simulink model "comp_hyb1206"  (R2018a)
settings: Solver=ode45  StartTime=0.0  StopTime=10  RelTol=1e-3  EnableMultiTasking=on
undefined symbols (not defined in the file or in its folder): Ion, Lithium, sigbuilder_block
libraries: powerlib x26, powerlib_meascontrol x7, powerlib_extras x2, electricdrivelib x1, re_lib x1
settings Model: Creator=Amr Saleh  LastModifiedBy=CC
settings DataIOCC: LimitDataPoints=on  SaveFormat=Array
settings OptimizationCC: LifeSpan=inf
settings DebuggingCC: SolverPrmCheckMsg=warning  SFUnexpectedBacktrackingDiag=warning  SFNoUnconditionalDefaultTransitionDiag=warning  SFExecutionAtInitializationDiag=none
settings HardwareCC: ProdBitPerPointer=32  ProdBitPerSizeT=32  ProdBitPerPtrDiffT=32  ProdLargestAtomicFloat=None  ProdIntDivRoundTo=Undefined  ProdEndianess=Unspecified  ProdWordSize=32  ProdHWDeviceType=32-bit Generic
settings ModelReferenceCC: PropagateSignalLabelsOutOfModel=off
settings CodeAppCC: StateflowObjectComments=on
settings GRTTargetCC: TargetLangStandard=C89/C90 (ANSI)  GeneratePreprocessorConditionals=Disable all
settings ConfigComp: CovMetricSettings=dw  CovHtmlReporting=on  CovSaveCumulativeToWorkspaceVar=on  CovSaveSingleToWorkspaceVar=on  CovExternalEMLEnable=off  CovSFcnEnable=off

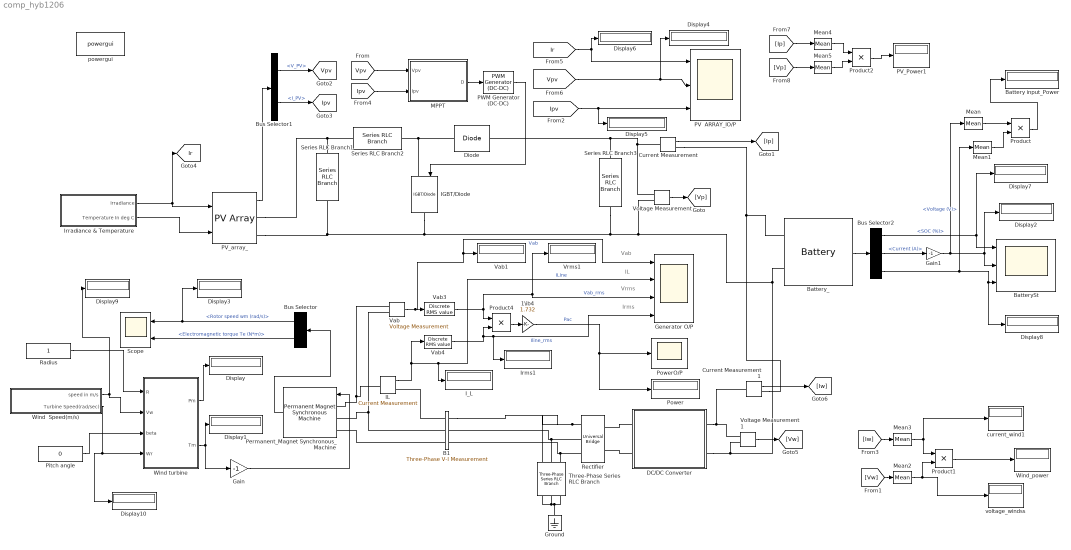
== system comp_hyb1206 ==
  note: Vrms
  note: Vab
  note: IL
  note: Irms
  1\ib4 : Gain  Gain=1.732  SaturateOnIntegerOverflow=on  OutDataTypeStr=Inherit: Same as input  ParamDataTypeStr=Inherit: Same as input
  B1 : powerlib/Measurements/Three-Phase V-I Measurement  VoltageMeasurement=phase-to-ground  SetLabelV=on  LabelV=Vabc_B1  Vpu=off  VpuLL=off  CurrentMeasurement=yes  SetLabelI=on  LabelI=Iabc_B1  Ipu=off  Pbase=100e6  Vbase=500e3  OutputType=Magnitude  PhasorSimulation=off  PSBequivalent=0
  Battery input_Power : Display
  BatterySt : Scope  NumInputPorts=3
  Battery_ : electricdrivelib/Extra Sources/Battery  BatType=Lithium-Ion  ShowTempParam=off  ThermalPreset=no  ShowAgeParam=off  NomV=240  NomQ=100  SOC=49.001  Batt_Tr=30  PresetModel=on  MaxQ=100  MinV=180  FullV=279.3569  Dis_rate=43.4783  R=0.024  Normal_OP=90.4348  expZone="[259.2926      4.913043]"  current=[6.5 13 32.5]  Units=Time  Tci=20  NomT=20  T2=-30  MaxQ2=4.8  FullV2=7.1  Normal_OP2=5.655  expZone2="[6.58           1]"  Rca=0.6  ti=2000  Dp=0  Neq0=0  Tsim=1e6  Ta1=25  Qeol=5.4*0.9  Reol=0.013333*1.2  Char_age=[2.3478, 3]  Dis_age=[2.3478, 10]  N1=1500  N2=10500  N3=1000  N4=1400  Ta2=45  N5=950
  Bus Selector : BusSelector  OutputSignals=Rotor speed wm (rad/s),Electromagnetic torque Te (N*m)
  Bus Selector1 : BusSelector  OutputSignals=V_PV,I_PV
  Bus Selector2 : BusSelector  OutputSignals=SOC (%),Current (A),Voltage (V)
  Current Measurement : powerlib/Measurements/Current Measurement  PhasorSimulation=off  OutputType=Complex  PSBequivalent=0
  Current Measurement1 : powerlib/Measurements/Current Measurement  PhasorSimulation=off  OutputType=Complex  PSBequivalent=0
  DC/DC Converter : Subsystem
  Diode : powerlib/Power Electronics/Diode  Ron=0.001  Lon=0  Vf=0.8  IC=0  UseSnubber=0  Rs=500  Cs=250e-9  Measurements=off
  Display{,1..10} (11 alike) : Display
      Display10 settings: Decimation=2
  Gain : Gain  Gain=-1
  Gain1 : Gain  Gain=-1
  Generator O/P : Scope  NumInputPorts=4
  Ground : powerlib/Elements/Ground  LConnTagsString=a
  IGBT/Diode : powerlib/Power Electronics/IGBT//Diode  Ron=1e-3  Rs=1e5  Cs=inf  Measurements=off
  IL : powerlib/Measurements/Current Measurement  PhasorSimulation=off  OutputType=Complex  PSBequivalent=0
  I_L : Display
      settings: SampleTime=1e-3
  Irms1 : Display
      settings: SampleTime=1e-3
  Irradiance & Temperature : Subsystem  Tag=STV Subsys  LoadFcn=sigbuilder_block('load');  StartFcn=sigbuilder_block('start');  StopFcn=sigbuilder_block('stop');  ClipboardFcn=sigbuilder_block('clipboard');  mask(Sigbuilder block){tuvar=[0:10]}
      mask help: Simulink:masks:SigbuilderBlock_MD
      mask init:
      | if ~strcmp(get_param(bdroot(gcbh),'SimulationStatus'),'stopped') tuvar = sigbuilder_block('maskInit'); end
      settings: CopyFcn=sigbuilder_block('copy');  DeleteFcn=sigbuilder_block('delete');  ModelCloseFcn=sigbuilder_block('modelClose');  PreSaveFcn=sigbuilder_block('preSave');  PauseFcn=sigbuilder_block('pause');  ContinueFcn=sigbuilder_block('continue');  NameChangeFcn=sigbuilder_block('namechange');  OpenFcn=sigbuilder_block('open',[437.4 186 550.8 400.2 ]);  CloseFcn=sigbuilder_block('close');
      mask Display: plot(0, 0, 100, 100,[2, 2, 32, 32, 2], [68, 8, 8, 68, 68],[32, 2], [38, 38], [32, 19, 2],[53, 60, 44], [32, 17, 17, 2],[16, 16, 31, 31]);txt = getActiveGroup(gcbh);text(2, 100, txt,'verticalAlignment', 'top');
  MPPT : MATLAB Function  TreatAsAtomicUnit=on
  Mean{,1..5} (6 alike) : powerlib_meascontrol/Measurements/Mean  Freq=60  Vinit=0  Ts=0
  PV  ARRAY_lO/P : Scope  NumInputPorts=3
  PV_Power1 : Display
  PV_array_ : re_lib/Solar/PV Array  Npar=2  Nser=5  PlotType=array @ 1000 W/m2 & specified temperatures  S_vec="[ 1000  500  100 ]"  Temp_C_vec="[ 45 25  ]"  ModuleName=User-defined  PlotWhenSelected=off  Pm=200.112  Ncell=60  Voc=32.9  Isc=8.21  Vm=26.4  Im=7.58  beta_Voc_pc=-0.35339  alpha_Isc_pc=0.055349  beta_Voc=-0.11627  alpha_Isc=0.0045442  IL=8.232  I0=2.1756e-10  nI=0.87743  Rsh=123.7196  Rs=0.3317  BAL=on  Tc=1e-6  Tfilter=5e-5
  PWM Generator (DC-DC) : powerlib_meascontrol/Pulse & Signal Generators/PWM Generator (DC-DC)  Fsw=5000  Ts=10e-6
  Permanent_Magnet Synchronous_Machine : powerlib/Machines/Permanent Magnet Synchronous Machine  NbPhases=3  FluxDistribution=Sinusoidal  RotorType=Round  MechanicalLoad=Torque Tm  PresetModel=No  ShowDetailedParameters=on  MeasurementBus=off  Resistance=0.0485  Inductance=8.5e-3  dqInductances=[8.5e-3,8.5e-3]  La=0.000395  MachineConstant=Flux linkage established by magnets (V.s)  Flux=0.433  VoltageCst=392.6876  TorqueCst=3.2475  Flat=120  Mechanical=[0.01197 0.001189 5]  PolePairs=4  InitialConditions=[0,0, 0,0]  InitialConditions5ph=[0 0 0 0 0 0]  TsPowergui=0  TsBlock=-1  RefAngle=90 degrees behind phase A axis (modified Park)
      settings: SourceProductName=Simscape Power Systems
  Pitch angle : Constant  Value=0
  Power : Display
      settings: SampleTime=1e-3
  PowerO/P : Scope
  Product : Product
  Product1 : Product
  Product2 : Product
  Product4 : Product  RndMeth=Zero
  Radius : Constant
  Rectifier : powerlib/Power Electronics/Universal Bridge  Arms=3  SnubberResistance=1e5  SnubberCapacitance=inf  Device=Diodes  Ron=1e-3  Lon=0  ForwardVoltages="[  0  0  ]"  ForwardVoltage=0  GTOparameters=[ 10e-6 , 20e-6 ]  IGBTparameters=[ 1e-6 , 2e-6 ]  Measurements=None  Measurements_2=None  converterType=Rectifier
  Scope : Scope  NumInputPorts=2
  Series RLC Branch1 : powerlib/Elements/Series RLC Branch  LConnTagsString=__new0  RConnTagsString=__new0  BranchType=RC  Resistance=1e-4  Inductance=1e-3  SetiL0=off  InitialCurrent=0  Capacitance=100e-6  Setx0=off  InitialVoltage=0  Measurements=None
  Series RLC Branch2 : powerlib/Elements/Series RLC Branch  LConnTagsString=__new0  RConnTagsString=__new0  BranchType=RL  Resistance=0.1  Inductance=5e-3  SetiL0=off  InitialCurrent=0  Capacitance=100e-6  Setx0=off  InitialVoltage=0  Measurements=None
  Series RLC Branch3 : powerlib/Elements/Series RLC Branch  LConnTagsString=__new0  RConnTagsString=__new0  BranchType=RC  Resistance=1e-4  Inductance=1e-3  SetiL0=off  InitialCurrent=0  Capacitance=3300e-6  Setx0=off  InitialVoltage=0  Measurements=None
  Three-Phase Series RLC Branch : powerlib/Elements/Three-Phase Series RLC Branch  LConnTagsString=A|B|C  RConnTagsString=A|B|C  BranchType=C  Resistance=25  Inductance=1e-3  Capacitance=10e-6  Measurements=None
  Vab : powerlib/Measurements/Voltage Measurement  PhasorSimulation=off  OutputType=Complex  PSBequivalent=0
  Vab1 : Display
      settings: SampleTime=1e-3
  Vab3 : powerlib_extras/Discrete Measurements/Discrete  RMS value  Freq=50  Mag_Init=0  Ts=20e-6
  Vab4 : powerlib_extras/Discrete Measurements/Discrete  RMS value  Freq=50  Mag_Init=0  Ts=20e-6
  Voltage Measurement : powerlib/Measurements/Voltage Measurement  PhasorSimulation=off  OutputType=Complex  PSBequivalent=0
  Voltage Measurement1 : powerlib/Measurements/Voltage Measurement  PhasorSimulation=off  OutputType=Complex  PSBequivalent=0
  Vrms1 : Display
      settings: SampleTime=1e-3
  Wind  Speed(m/s) : Subsystem  Tag=STV Subsys  LoadFcn=sigbuilder_block('load');  StartFcn=sigbuilder_block('start');  StopFcn=sigbuilder_block('stop');  ClipboardFcn=sigbuilder_block('clipboard');  mask(Sigbuilder block){tuvar=[0:10]}
      mask help: Simulink:masks:SigbuilderBlock_MD
      mask init:
      | if ~strcmp(get_param(bdroot(gcbh),'SimulationStatus'),'stopped') tuvar = sigbuilder_block('maskInit'); end
      settings: CopyFcn=sigbuilder_block('copy');  DeleteFcn=sigbuilder_block('delete');  ModelCloseFcn=sigbuilder_block('modelClose');  PreSaveFcn=sigbuilder_block('preSave');  PauseFcn=sigbuilder_block('pause');  ContinueFcn=sigbuilder_block('continue');  NameChangeFcn=sigbuilder_block('namechange');  OpenFcn=sigbuilder_block('open',[330.6 139.8 550.8 400.2 ]);  CloseFcn=sigbuilder_block('close');
      mask Display: plot(0, 0, 100, 100,[2, 2, 32, 32, 2], [68, 8, 8, 68, 68],[32, 2], [38, 38], [32, 19, 2],[53, 60, 44], [32, 17, 17, 2],[16, 16, 31, 31]);txt = getActiveGroup(gcbh);text(2, 100, txt,'verticalAlignment', 'top');
  Wind turbine : Subsystem
  Wind_power : Display
  current_wind1 : Display
  powergui : powerlib/powergui  Priority=1  SimulationMode=Discrete  SampleTime=1e-6  frequency=60  Iterations=50  frequencyindice=0  Pbase=100e6  ErrMax=1e-4  UnitsV=kV  UnitsW=MW  buscounter=0  FunctionMessages=off  echomessages=off  EnableUseOfTLC=off  CurrentSourceSwitches=off  DisableSnubberDevices=off  DisableRonSwitches=off  DisableVfSwitches=off  DisplayEquations=off  SolverType=Tustin/Backward Euler (TBE)  Interpol=off  ExternalGateDelay=off  methode=off  Ts=100  x0status=blocks  SPID=on  SwTol=0  HookPort=off  RestoreLinks=warning  ResistiveCurrentMeasurement=off  Frange=[0:2:500]  Ylog=off  Xlog=on  ShowGrid=off  save=off  variable=ZData  structure=0  ZoomFFT=off  StartTime=0.0  cycles=1  DisplayStyle=1  fundamental=60  FreqAxis=off  MaxFrequency=1000  frequencyindicesteady=1  RmsSteady=1  display=off
  voltage_windss : Display
  tag scope: Ipv=global, Ir=global, Vpv=global
  wires:
  Radius/1 -> Wind turbine/1(R)
  Wind  Speed(m/s)/1(speed in m/s) -> Display9/1, Wind turbine/2(Vw)
  Pitch angle/1 -> Wind turbine/3(beta)
  Wind  Speed(m/s)/2(Turbine Speed(rad/sec)) -> Display10/1, Wind turbine/4(Wr)
  Wind turbine/1(Pm) -> Display/1
  Vab4/1 -> Product4/2, Irms1/1, Generator O/P/4  "Iline_rms"
  1\ib4/1 -> Power/1, PowerO/P/1  "Pac"
  Product4/1 -> 1\ib4/1
  IL/1 -> I_L/1, Generator O/P/2, Vab4/1  "ILine"
  Vab/1 -> Vab1/1, Generator O/P/1, Vab3/1  "Vab"
  Vab3/1 -> Vrms1/1, Generator O/P/3, Product4/1  "Vab_rms"
  Wind turbine/2(Tm) -> Gain/1, Display1/1
  Gain/1 -> Permanent_Magnet Synchronous_Machine/1
  Permanent_Magnet Synchronous_Machine/1 -> Bus Selector/1
  Bus Selector/1 -> Display3/1, Scope/1  "<Rotor speed wm (rad/s)>"
  Bus Selector/2 -> Scope/2  "<Electromagnetic torque Te (N*m)>"
  [Vpv] -> MPPT/1(Vpv)
  Bus Selector1/2 -> [Ipv]  "<I_PV>"
  [Vpv] -> Display4/1, PV  ARRAY_lO/P/2
  PV_array_/1 -> Bus Selector1/1
  PWM Generator (DC-DC)/1 -> IGBT/Diode/1
  Bus Selector1/1 -> [Vpv]  "<V_PV>"
  MPPT/1(D) -> PWM Generator (DC-DC)/1
  [Ipv] -> Display5/1, PV  ARRAY_lO/P/3
  [Ipv] -> MPPT/2(Ipv)
  Battery_/1 -> Bus Selector2/1
  Bus Selector2/1 -> BatterySt/1, Display7/1  "<SOC (%)>"
  Bus Selector2/2 -> Gain1/1  "<Current (A)>"
  Bus Selector2/3 -> Mean1/1, Display8/1, BatterySt/3  "<Voltage (V)>"
  [Ir] -> PV  ARRAY_lO/P/1, Display6/1
  Gain1/1 -> Mean/1, Display2/1, BatterySt/2
  Mean/1 -> Product/1
  Mean1/1 -> Product/2
  Product/1 -> Battery input_Power/1
  Voltage Measurement/1 -> [Vp]
  Current Measurement/1 -> [Ip]
  [Ip] -> Mean4/1
  [Vp] -> Mean5/1
  Mean4/1 -> Product2/1
  Mean5/1 -> Product2/2
  Product2/1 -> PV_Power1/1
  Voltage Measurement1/1 -> [Vw]
  Current Measurement1/1 -> [Iw]
  [Vw] -> Mean2/1
  [Iw] -> Mean3/1
  Mean3/1 -> current_wind1/1, Product1/1
  Mean2/1 -> Product1/2, voltage_windss/1
  Product1/1 -> Wind_power/1
  Irradiance & Temperature/2(Temperature In deg C) -> PV_array_/2
  Irradiance & Temperature/1(Irradiance) -> PV_array_/1, [Ir]
  connections:
  Vab/LConn2 -- Permanent_Magnet Synchronous_Machine/LConn2 -- B1/LConn2
  Vab/LConn1 -- Permanent_Magnet Synchronous_Machine/LConn1 -- IL/LConn1
  B1/LConn1 -- IL/RConn1
  Rectifier/LConn1 -- B1/RConn1 -- Three-Phase Series RLC Branch/LConn1
  B1/LConn3 -- Permanent_Magnet Synchronous_Machine/LConn3
  Three-Phase Series RLC Branch/LConn3 -- B1/RConn3 -- Rectifier/LConn3
  Three-Phase Series RLC Branch/LConn2 -- B1/RConn2 -- Rectifier/LConn2
  Three-Phase Series RLC Branch/RConn3 -- Three-Phase Series RLC Branch/RConn1 -- Three-Phase Series RLC Branch/RConn2 -- Ground/LConn1
  Diode/LConn1 -- Series RLC Branch2/RConn1 -- IGBT/Diode/LConn1
  PV_array_/RConn1 -- Series RLC Branch2/LConn1 -- Series RLC Branch1/LConn1
  DC/DC Converter/LConn1 -- Rectifier/RConn1
  DC/DC Converter/LConn2 -- Rectifier/RConn2
  DC/DC Converter/RConn1 -- Voltage Measurement1/LConn1 -- Current Measurement1/LConn1
  Series RLC Branch3/RConn1 -- IGBT/Diode/RConn1 -- Series RLC Branch1/RConn1 -- PV_array_/RConn2 -- Voltage Measurement/LConn2 -- Voltage Measurement1/LConn2 -- DC/DC Converter/RConn2 -- Battery_/LConn2
  Series RLC Branch3/LConn1 -- Voltage Measurement/LConn1 -- Current Measurement/LConn1 -- Diode/RConn1
  Current Measurement/RConn1 -- Current Measurement1/RConn1 -- Battery_/LConn1

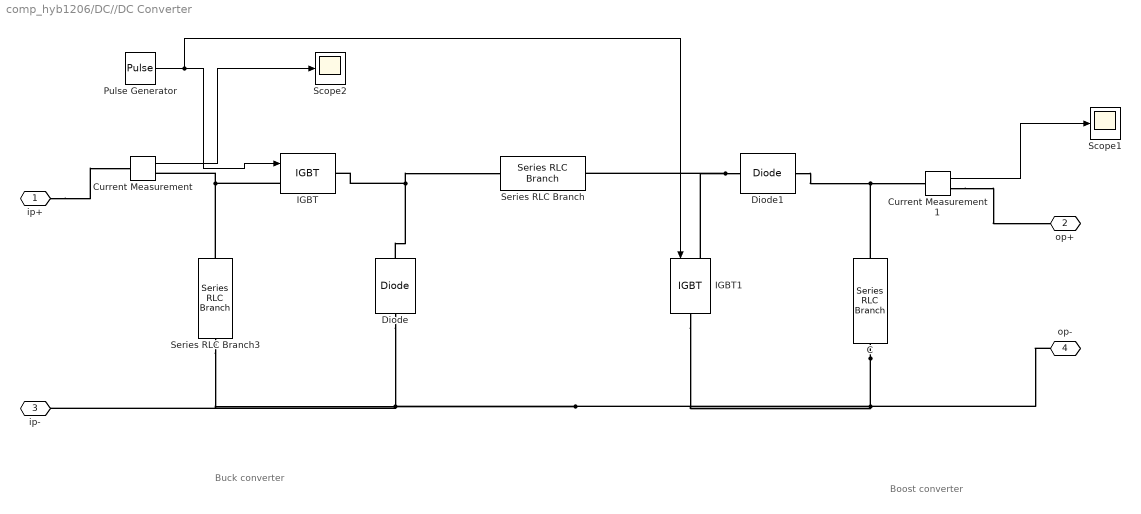
== system comp_hyb1206/DC//DC Converter ==
  note: Boost converter
  note: Buck converter
  C : powerlib/Elements/Series RLC Branch  LConnTagsString=__new0  RConnTagsString=__new0  BranchType=C  Resistance=1  Inductance=1e-3  SetiL0=off  InitialCurrent=0  Capacitance=32e-6  Setx0=off  InitialVoltage=0  Measurements=None
  Current Measurement : powerlib/Measurements/Current Measurement  PhasorSimulation=off  OutputType=Complex  PSBequivalent=0
  Current Measurement1 : powerlib/Measurements/Current Measurement  PhasorSimulation=off  OutputType=Complex  PSBequivalent=0
  Diode : powerlib/Power Electronics/Diode  Ron=0.0001  Lon=0  Vf=0.1  IC=0  UseSnubber=off  Rs=500  Cs=250e-9  Measurements=off
  Diode1 : powerlib/Power Electronics/Diode  Ron=0.0001  Lon=0  Vf=0.5  IC=0  UseSnubber=off  Rs=500  Cs=250e-9  Measurements=off
  IGBT : powerlib/Power Electronics/IGBT  Ron=0.0001  Lon=0  Vf=0.1  Tf=1e-6  Tt=2e-6  IC=0  Rs=1e5  Cs=inf  Measurements=off
  IGBT1 : powerlib/Power Electronics/IGBT  Ron=0.0001  Lon=0  Vf=0.5  Tf=1e-6  Tt=2e-6  IC=0  Rs=1e5  Cs=inf  Measurements=off
  Pulse Generator : DiscretePulseGenerator  PulseType=Time based  Period=1/5000  PulseWidth=80
  Scope1 : Scope
  Scope2 : Scope
  Series RLC Branch : powerlib/Elements/Series RLC Branch  LConnTagsString=__new0  RConnTagsString=__new0  BranchType=L  Resistance=1  Inductance=32e-3  SetiL0=off  InitialCurrent=0  Capacitance=1e-6  Setx0=off  InitialVoltage=0  Measurements=None
  Series RLC Branch3 : powerlib/Elements/Series RLC Branch  LConnTagsString=__new0  RConnTagsString=__new0  BranchType=C  Resistance=1  Inductance=1e-3  SetiL0=off  InitialCurrent=0  Capacitance=6700e-6  Setx0=off  InitialVoltage=0  Measurements=None
  ip+ : PMIOPort  Side=Left
  op+ : PMIOPort  Port=2  Side=Right
  ip- : PMIOPort  Port=3  Side=Left
  op- : PMIOPort  Port=4  Side=Right
  wires:
  Current Measurement1/1 -> Scope1/1
  Current Measurement/1 -> Scope2/1
  Pulse Generator/1 -> IGBT1/1, IGBT/1
  connections:
  Diode1/RConn1 -- C/RConn1 -- Current Measurement1/LConn1
  Diode1/LConn1 -- Series RLC Branch/RConn1 -- IGBT1/LConn1
  Diode/RConn1 -- Series RLC Branch/LConn1 -- IGBT/RConn1
  Current Measurement1/RConn1 -- op+/RConn1
  IGBT/LConn1 -- Series RLC Branch3/RConn1 -- Current Measurement/RConn1
  ip+/RConn1 -- Current Measurement/LConn1
  C/LConn1 -- IGBT1/RConn1 -- ip-/RConn1 -- Series RLC Branch3/LConn1 -- Diode/LConn1 -- op-/RConn1

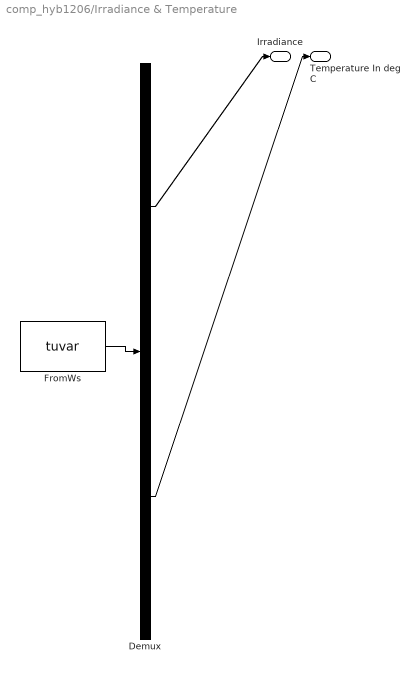
== system comp_hyb1206/Irradiance & Temperature ==
  Demux : Demux  Tag=STV Demux  Outputs=2
  FromWs : FromWorkspace  Tag=STV FromWs  VariableName=tuvar  SampleTime=0
      SigBuilderData=|
      | common.afterFinalStr = 'Extrapolate'
      | common.sampleTime = 0
      | dataSet.timeRange = [0 10]
      | dataSet.name = 'Group 1'
      | sbobj.Groups.Name = 'Group 1'
      | sbobj.Groups.Signals(1).Name = 'Irradiance'
      | sbobj.Groups.Signals(1).XData = [0 1 2 3 4 5 6 7 8 9 10]
      | sbobj.Groups.Signals(1).YData = [479.77 479.77 677.52 830.62 932.02 945.27 904.4 798.17 635.35 435.02 228.08]
      | sbobj.Groups.Signals(2).Name = 'Temperature In deg C'
      | sbobj.Groups.Signals(2).XData = [0 1 2 3 4 5 6 7 8 9 10]
      | sbobj.Groups.Signals(2).YData = [33.41 33.41 36.94 39.58 41.26 42.55 43.5 43.98 43.88 43.29 42.17]
  Irradiance : Outport  Tag=STV Outport
  Temperature In deg C : Outport  Tag=STV Outport  Port=2
  wires:
  FromWs/1 -> Demux/1
  Demux/1 -> Irradiance/1
  Demux/2 -> Temperature In deg C/1

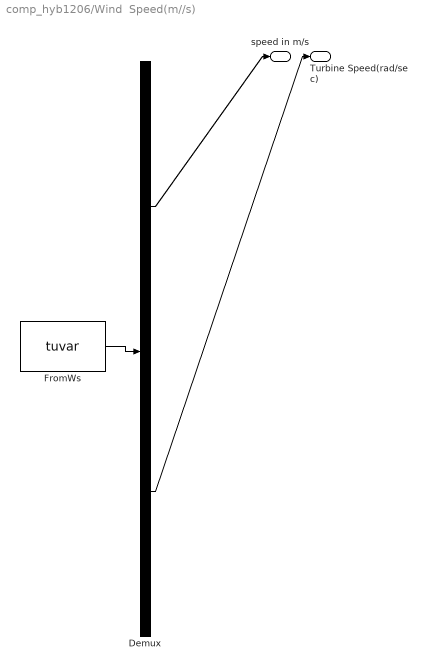
== system comp_hyb1206/Wind  Speed(m//s) ==
  Demux : Demux  Tag=STV Demux  Outputs=2
  FromWs : FromWorkspace  Tag=STV FromWs  VariableName=tuvar  SampleTime=0
      SigBuilderData=|
      | common.afterFinalStr = 'Extrapolate'
      | common.sampleTime = 0
      | dataSet.timeRange = [0 10]
      | dataSet.name = 'Group 1'
      | sbobj.Groups.Name = 'Group 1'
      | sbobj.Groups.Signals(1).Name = 'speed in m/s'
      | sbobj.Groups.Signals(1).XData = [0 1 2 3 4 5 6 7 8 9 10]
      | sbobj.Groups.Signals(1).YData = [10 10 10.4 12.4 11 12.4 9.2 9.6 13 11.6 13.3]
      | sbobj.Groups.Signals(2).Name = 'Turbine Speed(rad/sec)'
      | sbobj.Groups.Signals(2).XData = [0 1 2 3 4 5 6 7 8 9 10]
      | sbobj.Groups.Signals(2).YData = [66.9034 66.9034 69.5795 82.9602 73.5937 82.9602 61.5511 64.2273 86.9744 77.6079 88.9815]
  speed in m/s : Outport  Tag=STV Outport
  Turbine Speed(rad/sec) : Outport  Tag=STV Outport  Port=2
  wires:
  FromWs/1 -> Demux/1
  Demux/1 -> speed in m/s/1
  Demux/2 -> Turbine Speed(rad/sec)/1

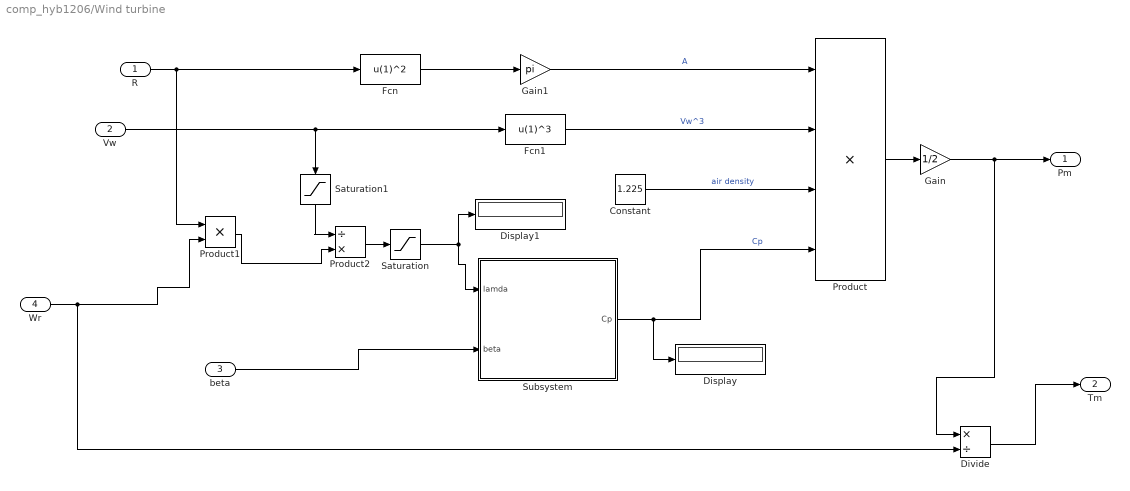
== system comp_hyb1206/Wind turbine ==
  R : Inport
  Vw : Inport  Port=2
  beta : Inport  Port=3
  Wr : Inport  Port=4
  Constant : Constant  Value=1.225
  Display : Display
  Display1 : Display
  Divide : Product  Inputs=*/
  Fcn : Fcn  Expr=u(1)^2
  Fcn1 : Fcn  Expr=u(1)^3
  Gain : Gain  Gain=1/2
  Gain1 : Gain  Gain=pi
  Product : Product  Inputs=4
  Product1 : Product
  Product2 : Product  Inputs=/*
  Saturation : Saturate  UpperLimit=inf  LowerLimit=1e-6
  Saturation1 : Saturate  UpperLimit=inf  LowerLimit=1e-6
  Subsystem : Subsystem
  Pm : Outport
  Tm : Outport  Port=2
  wires:
  Gain1/1 -> Product/1  "A"
  Fcn1/1 -> Product/2  "Vw^3"
  Constant/1 -> Product/3  "air density"
  Subsystem/1(Cp) -> Display/1, Product/4  "Cp"
  Gain/1 -> Divide/1, Pm/1
  Product/1 -> Gain/1
  Fcn/1 -> Gain1/1
  R/1 -> Fcn/1, Product1/1
  Vw/1 -> Fcn1/1, Saturation1/1
  beta/1 -> Subsystem/2(beta)
  Wr/1 -> Divide/2, Product1/2
  Product1/1 -> Product2/2
  Product2/1 -> Saturation/1
  Saturation/1 -> Subsystem/1(lamda), Display1/1
  Saturation1/1 -> Product2/1
  Divide/1 -> Tm/1

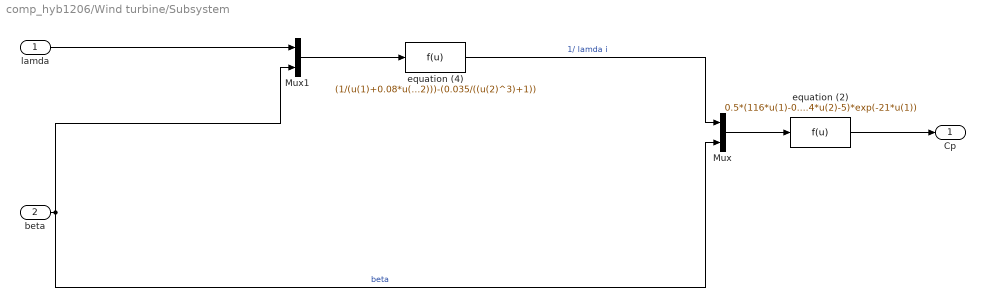
== system comp_hyb1206/Wind turbine/Subsystem ==
  lamda : Inport
  beta : Inport  Port=2
  Mux : Mux  Inputs=2
  Mux1 : Mux  Inputs=2
  equation (2) : Fcn  Expr=0.5*(116*u(1)-0.4*u(2)-5)*exp(-21*u(1))
  equation (4) : Fcn  Expr=(1/(u(1)+0.08*u(2)))-(0.035/((u(2)^3)+1))
  Cp : Outport
  wires:
  equation (2)/1 -> Cp/1
  Mux/1 -> equation (2)/1
  equation (4)/1 -> Mux/1  "1/ lamda i"
  beta/1 -> Mux/2, Mux1/2  "beta"
  Mux1/1 -> equation (4)/1
  lamda/1 -> Mux1/1

== matlab function comp_hyb1206/MPPT ==
  data: Vpv input; D output; Ipv input
function D = Pand0(Vpv,Ipv)



persistent Dprev Pprev Vprev

if isempty (Dprev) 
   
Dprev = 0.7;

Vprev = 190;

Pprev = 2000;

end

deltaD = 125e-6;

% Calculate measured array power

Ppv = Vpv*Ipv;

% Increase or decrease duty cycle based on conditions

if (Ppv-Pprev) ~= 0 
    if (Ppv-Pprev) > 0

if (Vpv-Vprev) > 0

D= Dprev - deltaD;

else

D = Dprev + deltaD;

end

else

if (Vpv-Vprev) > 0

D= Dprev + deltaD;

else

D = Dprev - deltaD;

end
    end
else
    D = Dprev;
end
% Update internal values

Dprev = D;

Vprev = Vpv; 

Pprev = Ppv;
